simulink model "pend_cart"  (R2018a)
settings: Solver=ode5  StartTime=0.0  StopTime=inf  FixedStep=Ts  RelTol=1e-3
model workspace (MAT data in the model file):
  t_sig = mpt.Signal
  t_sig.DataType = 'auto'
  t_sig.Dimensions = -1
  t_sig.DimensionsMode = 'auto'
  t_sig.Complexity = 'auto'
  t_sig.SampleTime = -1
  t_sig.SamplingMode = 'auto'
  u_sig = mpt.Signal
  u_sig.DataType = 'auto'
  u_sig.Dimensions = -1
  u_sig.DimensionsMode = 'auto'
  u_sig.Complexity = 'auto'
  u_sig.SampleTime = -1
  u_sig.SamplingMode = 'auto'
  y_sig = mpt.Signal
  y_sig.DataType = 'auto'
  y_sig.Dimensions = -1
  y_sig.DimensionsMode = 'auto'
  y_sig.Complexity = 'auto'
  y_sig.SampleTime = -1
  y_sig.SamplingMode = 'auto'
values from neighbouring files (symbols this model uses):
  X0 = Simulink.Parameter    [pend_init.m]    (also in test.m)
undefined symbols (not defined in the file or in its folder): X_d_0
settings Model: Creator=sam  LastModifiedBy=sam
settings OptimizationCC: DefaultParameterBehavior=Inlined  BufferReuse=off  GlobalBufferReuse=off  ExpressionFolding=off  EnableMemcpy=off  PassReuseOutputArgsAs=Individual arguments  LocalBlockOutputs=off  OptimizeDataStoreBuffers=off  BusAssignmentInplaceUpdate=off  OptimizationLevel=level0  OptimizationCustomize=off
settings DebuggingCC: MultiTaskCondExecSysMsg=warning  MultiTaskRateTransMsg=warning  ParameterTunabilityLossMsg=error
settings HardwareCC: TargetBitPerLong=64  TargetBitPerPointer=64  TargetBitPerSizeT=64  TargetBitPerPtrDiffT=64  TargetLongLongMode=on  TargetIntDivRoundTo=Zero  TargetEndianess=LittleEndian  TargetWordSize=64  TargetHWDeviceType=MATLAB Host  ProdEqTarget=off
settings SFSimCC: MATLABDynamicMemAlloc=off
settings RTWCC: SystemTargetFile=ert_shrlib.tlc  TemplateMakefile=ert_default_tmf  Description=Embedded Coder (host-based shared library target)  IncludeHyperlinkInReport=on
settings CodeAppCC: ForceParamTrailComments=on  IgnoreCustomStorageClasses=off  OperatorAnnotations=on  SimulinkDataObjDesc=on  SFDataObjDesc=on  InsertBlockDesc=on
settings STFCustomTargetCC: TargetLangStandard=C99 (ISO)  MultiwordLength=256  GenerateSampleERTMain=on  ParMdlRefBuildCompliant=on  CompOptLevelCompliant=on  CombineOutputUpdateFcns=on  ERTCustomFileBanners=on  SupportComplex=off  SupportNonInlinedSFcns=off  RemoveResetFunc=on  MATLABClassNameForMDSCustomization=Simulink.SoftwareTarget.ERTCustomization  ModelStepFunctionPrototypeControlCompliant=on  GRTInterface=off  UseToolchainInfoCompliant=on  SystemTargetFile=ert_shrlib.tlc
settings ERTTargetCC: TargetLangStandard=C99 (ISO)  GenerateSampleERTMain=on  ConcurrentExecutionCompliant=off  SupportComplex=off  SupportContinuousTime=on  CPPClassGenCompliant=off  InlinedParameterPlacement=NonHierarchical  ERTCustomFileTemplate=example_file_process.tlc

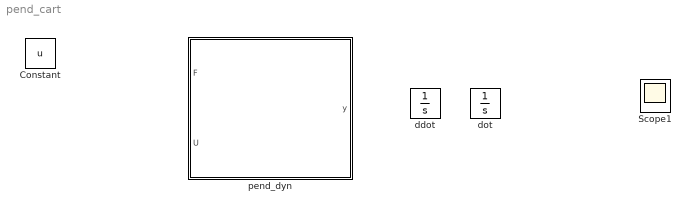
== system pend_cart ==
  Constant : Constant  Value=u
  Scope1 : Scope  NumInputPorts=2
  ddot : Integrator  InitialCondition=X_d_0
  dot : Integrator  InitialCondition=X0
  pend_dyn : MATLAB Function  TreatAsAtomicUnit=on

== matlab function pend_cart/pend_dyn ==
  data: F input; U input; y output size=2
function y = pend_dyn(F, U)
m = 1;
M = 1;
l = 1;
J = 1;
g = 9.8;
c = 1;
lam=1;
x = U(1)
theta = U(2)
x_dot = U(3)
theta_dot = U(4)
MM = (m+M)
jml= (J+m*l^2)
mlc = m*l*cos(theta)
mls = m*l*sin(theta)
MMatrix = [MM -mlc;-mlc jml]
MMatrix_inv = inv(MMatrix)
Fmat = [F;0]
dyn = [c*x_dot+mls*theta_dot^2;lam*theta_dot-g*mls]
y = MMatrix_inv*(Fmat-dyn)
end
